simulink model "Problem_3"  (R2020a)
settings: Solver=VariableStepAuto  StartTime=0.0  StopTime=10.0  RelTol=1e-3
settings Model: Creator=Ganesh  LastModifiedBy=Ganesh
settings DataIOCC: ExternalInput=[t, F]  SaveFormat=Structure

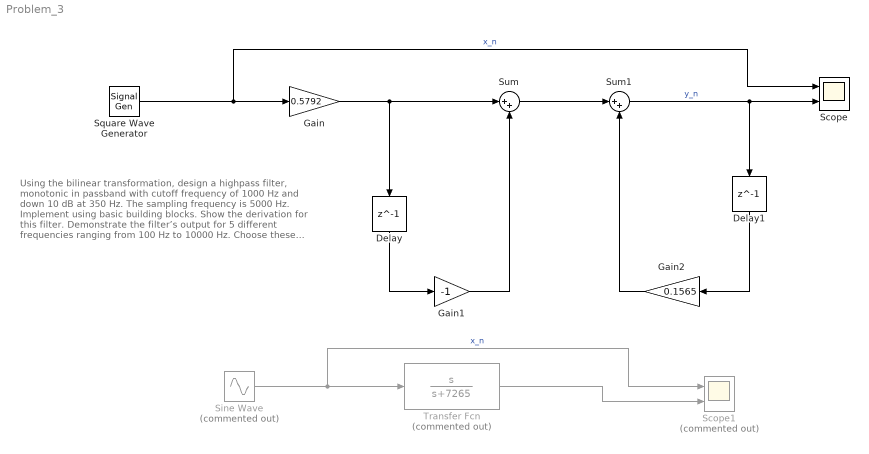
== system Problem_3 ==
  note: Using the bilinear transformation, design a highpass filter, monotonic in passband with cutoff frequency of 1000 Hz and down 10 dB at 350 Hz. The sampling frequency is 5000 Hz. Implement using basic building blocks. Show the derivation for this filter. Demonstrate the filter’s output for 5 different frequencies ranging from 100 Hz to 10000 Hz. Choose these frequencies smartly to demonstrate the filter working.
  Delay : Delay  DelayLength=1
  Delay1 : Delay  DelayLength=1
  Gain : Gain  Gain=0.5792
  Gain1 : Gain  Gain=-1
  Gain2 : Gain  Gain=0.1565
  Scope : Scope  NumInputPorts=2
  Scope1 : Scope  Commented=on  NumInputPorts=2
  Sine Wave : Sin  Commented=on  Frequency=5000*6.28  SampleTime=0
  Square Wave Generator : SignalGenerator  WaveForm=square  Frequency=7000
  Sum : Sum  Inputs=|++
  Sum1 : Sum  Inputs=|++
  Transfer Fcn : TransferFcn  Commented=on  Numerator=[1 0]  Denominator=[1 7265]
  wires:
  Square Wave Generator/1 -> Scope/1, Gain/1  "x_n"
  Gain/1 -> Delay/1, Sum/1
  Delay/1 -> Gain1/1
  Gain1/1 -> Sum/2
  Sum/1 -> Sum1/1
  Sum1/1 -> Delay1/1, Scope/2  "y_n"
  Delay1/1 -> Gain2/1
  Gain2/1 -> Sum1/2
  Sine Wave/1 -> Scope1/1, Transfer Fcn/1  "x_n"
  Transfer Fcn/1 -> Scope1/2
